simulink model "gm_parallel_min_cost_function_vopt_6phase"  (R2022a)
settings: Solver=FixedStepDiscrete  StartTime=0.0  StopTime=10.0  RelTol=1e-3
undefined symbols (not defined in the file or in its folder): f_c
libraries: hdlmdlgenlib x368
(part 3 of 3)

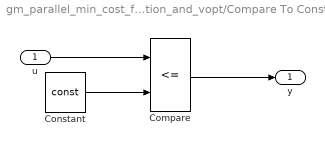
== system gm_parallel_min_cost_function_vopt_6phase/Min_cost_function_and_vopt/Compare To Constant ==
  u : Inport  OutDataTypeStr=int32  SampleTime=1e-08
  Compare : RelationalOperator  Operator=<=  OutDataTypeStr=boolean
  Constant : Constant  DisableCoverage=on  Value=const  OutDataTypeStr=Inherit: Inherit via back propagation  SampleTime=-1
  y : Outport  SampleTime=1e-08
  wires:
  u/1 -> Compare/1
  Compare/1 -> y/1
  Constant/1 -> Compare/2

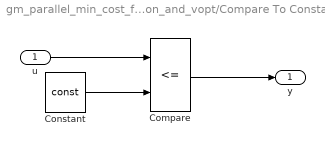
== system gm_parallel_min_cost_function_vopt_6phase/Min_cost_function_and_vopt/Compare To Constant1 ==
  u : Inport  OutDataTypeStr=fixdt(1, 33, 0)  SampleTime=1e-08
  Compare : RelationalOperator  Operator=<=  OutDataTypeStr=boolean
  Constant : Constant  DisableCoverage=on  Value=const  OutDataTypeStr=Inherit: Inherit via back propagation  SampleTime=-1
  y : Outport  SampleTime=1e-08
  wires:
  u/1 -> Compare/1
  Compare/1 -> y/1
  Constant/1 -> Compare/2

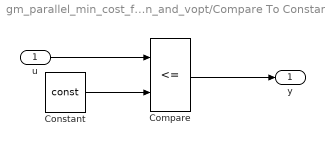
== system gm_parallel_min_cost_function_vopt_6phase/Min_cost_function_and_vopt/Compare To Constant10 ==
  u : Inport  OutDataTypeStr=fixdt(1, 33, 0)  SampleTime=1e-08
  Compare : RelationalOperator  Operator=<=  OutDataTypeStr=boolean
  Constant : Constant  DisableCoverage=on  Value=const  OutDataTypeStr=Inherit: Inherit via back propagation  SampleTime=-1
  y : Outport  SampleTime=1e-08
  wires:
  u/1 -> Compare/1
  Compare/1 -> y/1
  Constant/1 -> Compare/2

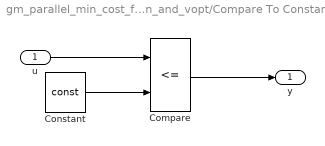
== system gm_parallel_min_cost_function_vopt_6phase/Min_cost_function_and_vopt/Compare To Constant11 ==
  u : Inport  OutDataTypeStr=fixdt(1, 33, 0)  SampleTime=1e-08
  Compare : RelationalOperator  Operator=<=  OutDataTypeStr=boolean
  Constant : Constant  DisableCoverage=on  Value=const  OutDataTypeStr=Inherit: Inherit via back propagation  SampleTime=-1
  y : Outport  SampleTime=1e-08
  wires:
  u/1 -> Compare/1
  Compare/1 -> y/1
  Constant/1 -> Compare/2

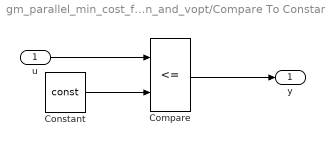
== system gm_parallel_min_cost_function_vopt_6phase/Min_cost_function_and_vopt/Compare To Constant12 ==
  u : Inport  OutDataTypeStr=fixdt(1, 33, 0)  SampleTime=1e-08
  Compare : RelationalOperator  Operator=<=  OutDataTypeStr=boolean
  Constant : Constant  DisableCoverage=on  Value=const  OutDataTypeStr=Inherit: Inherit via back propagation  SampleTime=-1
  y : Outport  SampleTime=1e-08
  wires:
  u/1 -> Compare/1
  Compare/1 -> y/1
  Constant/1 -> Compare/2

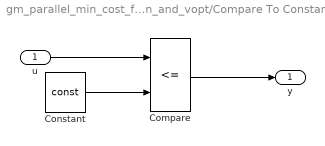
== system gm_parallel_min_cost_function_vopt_6phase/Min_cost_function_and_vopt/Compare To Constant13 ==
  u : Inport  OutDataTypeStr=fixdt(1, 33, 0)  SampleTime=1e-08
  Compare : RelationalOperator  Operator=<=  OutDataTypeStr=boolean
  Constant : Constant  DisableCoverage=on  Value=const  OutDataTypeStr=Inherit: Inherit via back propagation  SampleTime=-1
  y : Outport  SampleTime=1e-08
  wires:
  u/1 -> Compare/1
  Compare/1 -> y/1
  Constant/1 -> Compare/2

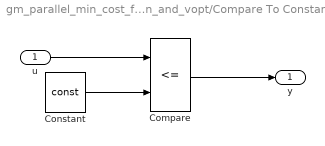
== system gm_parallel_min_cost_function_vopt_6phase/Min_cost_function_and_vopt/Compare To Constant14 ==
  u : Inport  OutDataTypeStr=fixdt(1, 33, 0)  SampleTime=1e-08
  Compare : RelationalOperator  Operator=<=  OutDataTypeStr=boolean
  Constant : Constant  DisableCoverage=on  Value=const  OutDataTypeStr=Inherit: Inherit via back propagation  SampleTime=-1
  y : Outport  SampleTime=1e-08
  wires:
  u/1 -> Compare/1
  Compare/1 -> y/1
  Constant/1 -> Compare/2

== system gm_parallel_min_cost_function_vopt_6phase/Min_cost_function_and_vopt/Compare To Constant15 ==
  u : Inport  OutDataTypeStr=fixdt(1, 33, 0)  SampleTime=1e-08
  Compare : RelationalOperator  Operator=<=  OutDataTypeStr=boolean
  Constant : Constant  DisableCoverage=on  Value=const  OutDataTypeStr=Inherit: Inherit via back propagation  SampleTime=-1
  y : Outport  SampleTime=1e-08
  wires:
  u/1 -> Compare/1
  Compare/1 -> y/1
  Constant/1 -> Compare/2

== system gm_parallel_min_cost_function_vopt_6phase/Min_cost_function_and_vopt/Compare To Constant2 ==
  u : Inport  OutDataTypeStr=fixdt(1, 33, 0)  SampleTime=1e-08
  Compare : RelationalOperator  Operator=<=  OutDataTypeStr=boolean
  Constant : Constant  DisableCoverage=on  Value=const  OutDataTypeStr=Inherit: Inherit via back propagation  SampleTime=-1
  y : Outport  SampleTime=1e-08
  wires:
  u/1 -> Compare/1
  Compare/1 -> y/1
  Constant/1 -> Compare/2

== system gm_parallel_min_cost_function_vopt_6phase/Min_cost_function_and_vopt/Compare To Constant3 ==
  u : Inport  OutDataTypeStr=fixdt(1, 33, 0)  SampleTime=1e-08
  Compare : RelationalOperator  Operator=<=  OutDataTypeStr=boolean
  Constant : Constant  DisableCoverage=on  Value=const  OutDataTypeStr=Inherit: Inherit via back propagation  SampleTime=-1
  y : Outport  SampleTime=1e-08
  wires:
  u/1 -> Compare/1
  Compare/1 -> y/1
  Constant/1 -> Compare/2

== system gm_parallel_min_cost_function_vopt_6phase/Min_cost_function_and_vopt/Compare To Constant4 ==
  u : Inport  OutDataTypeStr=fixdt(1, 33, 0)  SampleTime=1e-08
  Compare : RelationalOperator  Operator=<=  OutDataTypeStr=boolean
  Constant : Constant  DisableCoverage=on  Value=const  OutDataTypeStr=Inherit: Inherit via back propagation  SampleTime=-1
  y : Outport  SampleTime=1e-08
  wires:
  u/1 -> Compare/1
  Compare/1 -> y/1
  Constant/1 -> Compare/2

== system gm_parallel_min_cost_function_vopt_6phase/Min_cost_function_and_vopt/Compare To Constant5 ==
  u : Inport  OutDataTypeStr=fixdt(1, 33, 0)  SampleTime=1e-08
  Compare : RelationalOperator  Operator=<=  OutDataTypeStr=boolean
  Constant : Constant  DisableCoverage=on  Value=const  OutDataTypeStr=Inherit: Inherit via back propagation  SampleTime=-1
  y : Outport  SampleTime=1e-08
  wires:
  u/1 -> Compare/1
  Compare/1 -> y/1
  Constant/1 -> Compare/2

== system gm_parallel_min_cost_function_vopt_6phase/Min_cost_function_and_vopt/Compare To Constant6 ==
  u : Inport  OutDataTypeStr=fixdt(1, 33, 0)  SampleTime=1e-08
  Compare : RelationalOperator  Operator=<=  OutDataTypeStr=boolean
  Constant : Constant  DisableCoverage=on  Value=const  OutDataTypeStr=Inherit: Inherit via back propagation  SampleTime=-1
  y : Outport  SampleTime=1e-08
  wires:
  u/1 -> Compare/1
  Compare/1 -> y/1
  Constant/1 -> Compare/2

== system gm_parallel_min_cost_function_vopt_6phase/Min_cost_function_and_vopt/Compare To Constant7 ==
  u : Inport  OutDataTypeStr=fixdt(1, 33, 0)  SampleTime=1e-08
  Compare : RelationalOperator  Operator=<=  OutDataTypeStr=boolean
  Constant : Constant  DisableCoverage=on  Value=const  OutDataTypeStr=Inherit: Inherit via back propagation  SampleTime=-1
  y : Outport  SampleTime=1e-08
  wires:
  u/1 -> Compare/1
  Compare/1 -> y/1
  Constant/1 -> Compare/2

== system gm_parallel_min_cost_function_vopt_6phase/Min_cost_function_and_vopt/Compare To Constant8 ==
  u : Inport  OutDataTypeStr=fixdt(1, 33, 0)  SampleTime=1e-08
  Compare : RelationalOperator  Operator=<=  OutDataTypeStr=boolean
  Constant : Constant  DisableCoverage=on  Value=const  OutDataTypeStr=Inherit: Inherit via back propagation  SampleTime=-1
  y : Outport  SampleTime=1e-08
  wires:
  u/1 -> Compare/1
  Compare/1 -> y/1
  Constant/1 -> Compare/2

== system gm_parallel_min_cost_function_vopt_6phase/Min_cost_function_and_vopt/Compare To Constant9 ==
  u : Inport  OutDataTypeStr=fixdt(1, 33, 0)  SampleTime=1e-08
  Compare : RelationalOperator  Operator=<=  OutDataTypeStr=boolean
  Constant : Constant  DisableCoverage=on  Value=const  OutDataTypeStr=Inherit: Inherit via back propagation  SampleTime=-1
  y : Outport  SampleTime=1e-08
  wires:
  u/1 -> Compare/1
  Compare/1 -> y/1
  Constant/1 -> Compare/2

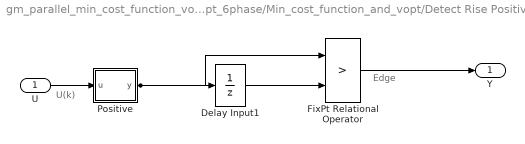
== system gm_parallel_min_cost_function_vopt_6phase/Min_cost_function_and_vopt/Detect Rise Positive ==
  note: Edge
  note: U(k)
  U : Inport  OutDataTypeStr=boolean  SampleTime=1e-08
  Delay Input1 : UnitDelay  Description=Store in Global RAM  DisableCoverage=on  InitialCondition=vinit  SampleTime=-1  HasFrameUpgradeWarning=on
  FixPt Relational Operator : RelationalOperator  Operator=>  OutDataTypeStr=boolean  ZeroCross=off  InputSameDT=off
  Positive : Subsystem  mask(Compare To Zero){relop=>, OutDataTypeStr=boolean, ZeroCross=off}
      mask prompts: relop "Simulink:masks:Operator_MP"; OutDataTypeStr "Simulink:masks:OutputDataType_MP"; ZeroCross "Simulink:masks:EnableZerocrossingDetection_MP"
      mask help: Simulink:masks:CompareToZero_MD
      mask init:
      | OutDataTypeStr = 'boolean';
      | ZeroCross = 'off';
      | blkName = 'parallel_min_cost_function_vopt_6phase/Min_cost_function_and_vopt/Detect Rise\nPositive/Positive';
      | relop = '>';
      | setValue = 'boolean';
      mask TypeOptions relop: == | ~= | < | <= | >= | >
      mask TypeOptions OutDataTypeStr: Simulink:masks:uint8 | Simulink:masks:boolean
      mask Callback ZeroCross: sl('zeroCrossEnable', gcbh);
      mask Display: disp([relop,' 0'])
  Y : Outport  SampleTime=1e-08
  wires:
  U/1 -> Positive/1(u)
  Delay Input1/1 -> FixPt Relational Operator/2
  FixPt Relational Operator/1 -> Y/1
  Positive/1(y) -> FixPt Relational Operator/1, Delay Input1/1

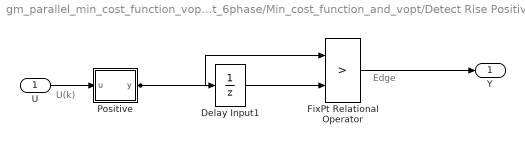
== system gm_parallel_min_cost_function_vopt_6phase/Min_cost_function_and_vopt/Detect Rise Positive1 ==
  note: Edge
  note: U(k)
  U : Inport  OutDataTypeStr=boolean  SampleTime=1e-08
  Delay Input1 : UnitDelay  Description=Store in Global RAM  DisableCoverage=on  InitialCondition=vinit  SampleTime=-1  HasFrameUpgradeWarning=on
  FixPt Relational Operator : RelationalOperator  Operator=>  OutDataTypeStr=boolean  ZeroCross=off  InputSameDT=off
  Positive : Subsystem  mask(Compare To Zero){relop=>, OutDataTypeStr=boolean, ZeroCross=off}
      mask prompts: relop "Simulink:masks:Operator_MP"; OutDataTypeStr "Simulink:masks:OutputDataType_MP"; ZeroCross "Simulink:masks:EnableZerocrossingDetection_MP"
      mask help: Simulink:masks:CompareToZero_MD
      mask init:
      | OutDataTypeStr = 'boolean';
      | ZeroCross = 'off';
      | blkName = 'parallel_min_cost_function_vopt_6phase/Min_cost_function_and_vopt/Detect Rise\nPositive1/Positive';
      | relop = '>';
      | setValue = 'boolean';
      mask TypeOptions relop: == | ~= | < | <= | >= | >
      mask TypeOptions OutDataTypeStr: Simulink:masks:uint8 | Simulink:masks:boolean
      mask Callback ZeroCross: sl('zeroCrossEnable', gcbh);
      mask Display: disp([relop,' 0'])
  Y : Outport  SampleTime=1e-08
  wires:
  U/1 -> Positive/1(u)
  Delay Input1/1 -> FixPt Relational Operator/2
  FixPt Relational Operator/1 -> Y/1
  Positive/1(y) -> FixPt Relational Operator/1, Delay Input1/1

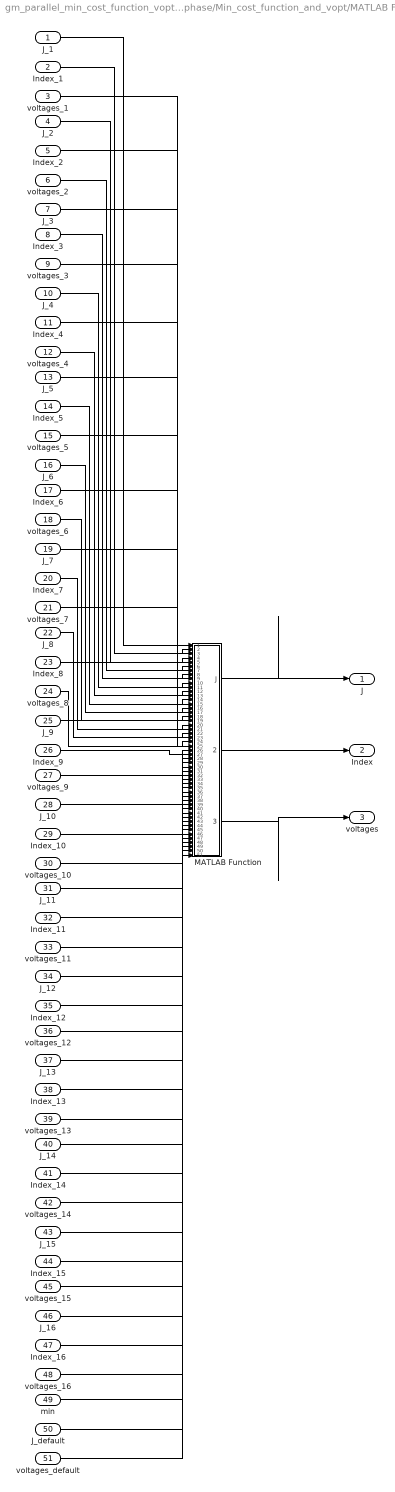
== system gm_parallel_min_cost_function_vopt_6phase/Min_cost_function_and_vopt/MATLAB Function ==
  J_1 : Inport  OutDataTypeStr=fixdt(1, 20, 11)  PortDimensions=1  SampleTime=1e-08
  Index_1 : Inport  Port=2  OutDataTypeStr=int32  PortDimensions=1  SampleTime=1e-08
  voltages_1 : Inport  Port=3  OutDataTypeStr=fixdt(1, 24, 11)  PortDimensions=[4]  SampleTime=1e-08
  J_2 : Inport  Port=4  OutDataTypeStr=fixdt(1, 20, 11)  PortDimensions=1  SampleTime=1e-08
  Index_2 : Inport  Port=5  OutDataTypeStr=int32  PortDimensions=1  SampleTime=1e-08
  voltages_2 : Inport  Port=6  OutDataTypeStr=fixdt(1, 24, 11)  PortDimensions=[4]  SampleTime=1e-08
  J_3 : Inport  Port=7  OutDataTypeStr=fixdt(1, 20, 11)  PortDimensions=1  SampleTime=1e-08
  Index_3 : Inport  Port=8  OutDataTypeStr=int32  PortDimensions=1  SampleTime=1e-08
  voltages_3 : Inport  Port=9  OutDataTypeStr=fixdt(1, 24, 11)  PortDimensions=[4]  SampleTime=1e-08
  J_4 : Inport  Port=10  OutDataTypeStr=fixdt(1, 20, 11)  PortDimensions=1  SampleTime=1e-08
  Index_4 : Inport  Port=11  OutDataTypeStr=int32  PortDimensions=1  SampleTime=1e-08
  voltages_4 : Inport  Port=12  OutDataTypeStr=fixdt(1, 24, 11)  PortDimensions=[4]  SampleTime=1e-08
  J_5 : Inport  Port=13  OutDataTypeStr=fixdt(1, 20, 11)  PortDimensions=1  SampleTime=1e-08
  Index_5 : Inport  Port=14  OutDataTypeStr=int32  PortDimensions=1  SampleTime=1e-08
  voltages_5 : Inport  Port=15  OutDataTypeStr=fixdt(1, 24, 11)  PortDimensions=[4]  SampleTime=1e-08
  J_6 : Inport  Port=16  OutDataTypeStr=fixdt(1, 20, 11)  PortDimensions=1  SampleTime=1e-08
  Index_6 : Inport  Port=17  OutDataTypeStr=int32  PortDimensions=1  SampleTime=1e-08
  voltages_6 : Inport  Port=18  OutDataTypeStr=fixdt(1, 24, 11)  PortDimensions=[4]  SampleTime=1e-08
  J_7 : Inport  Port=19  OutDataTypeStr=fixdt(1, 20, 11)  PortDimensions=1  SampleTime=1e-08
  Index_7 : Inport  Port=20  OutDataTypeStr=int32  PortDimensions=1  SampleTime=1e-08
  voltages_7 : Inport  Port=21  OutDataTypeStr=fixdt(1, 24, 11)  PortDimensions=[4]  SampleTime=1e-08
  J_8 : Inport  Port=22  OutDataTypeStr=fixdt(1, 20, 11)  PortDimensions=1  SampleTime=1e-08
  Index_8 : Inport  Port=23  OutDataTypeStr=int32  PortDimensions=1  SampleTime=1e-08
  voltages_8 : Inport  Port=24  OutDataTypeStr=fixdt(1, 24, 11)  PortDimensions=[4]  SampleTime=1e-08
  J_9 : Inport  Port=25  OutDataTypeStr=fixdt(1, 20, 11)  PortDimensions=1  SampleTime=1e-08
  Index_9 : Inport  Port=26  OutDataTypeStr=int32  PortDimensions=1  SampleTime=1e-08
  voltages_9 : Inport  Port=27  OutDataTypeStr=fixdt(1, 24, 11)  PortDimensions=[4]  SampleTime=1e-08
  J_10 : Inport  Port=28  OutDataTypeStr=fixdt(1, 20, 11)  PortDimensions=1  SampleTime=1e-08
  Index_10 : Inport  Port=29  OutDataTypeStr=int32  PortDimensions=1  SampleTime=1e-08
  voltages_10 : Inport  Port=30  OutDataTypeStr=fixdt(1, 24, 11)  PortDimensions=[4]  SampleTime=1e-08
  J_11 : Inport  Port=31  OutDataTypeStr=fixdt(1, 20, 11)  PortDimensions=1  SampleTime=1e-08
  Index_11 : Inport  Port=32  OutDataTypeStr=int32  PortDimensions=1  SampleTime=1e-08
  voltages_11 : Inport  Port=33  OutDataTypeStr=fixdt(1, 24, 11)  PortDimensions=[4]  SampleTime=1e-08
  J_12 : Inport  Port=34  OutDataTypeStr=fixdt(1, 20, 11)  PortDimensions=1  SampleTime=1e-08
  Index_12 : Inport  Port=35  OutDataTypeStr=int32  PortDimensions=1  SampleTime=1e-08
  voltages_12 : Inport  Port=36  OutDataTypeStr=fixdt(1, 24, 11)  PortDimensions=[4]  SampleTime=1e-08
  J_13 : Inport  Port=37  OutDataTypeStr=fixdt(1, 20, 11)  PortDimensions=1  SampleTime=1e-08
  Index_13 : Inport  Port=38  OutDataTypeStr=int32  PortDimensions=1  SampleTime=1e-08
  voltages_13 : Inport  Port=39  OutDataTypeStr=fixdt(1, 24, 11)  PortDimensions=[4]  SampleTime=1e-08
  J_14 : Inport  Port=40  OutDataTypeStr=fixdt(1, 20, 11)  PortDimensions=1  SampleTime=1e-08
  Index_14 : Inport  Port=41  OutDataTypeStr=int32  PortDimensions=1  SampleTime=1e-08
  voltages_14 : Inport  Port=42  OutDataTypeStr=fixdt(1, 24, 11)  PortDimensions=[4]  SampleTime=1e-08
  J_15 : Inport  Port=43  OutDataTypeStr=fixdt(1, 20, 11)  PortDimensions=1  SampleTime=1e-08
  Index_15 : Inport  Port=44  OutDataTypeStr=int32  PortDimensions=1  SampleTime=1e-08
  voltages_15 : Inport  Port=45  OutDataTypeStr=fixdt(1, 24, 11)  PortDimensions=[4]  SampleTime=1e-08
  J_16 : Inport  Port=46  OutDataTypeStr=fixdt(1, 20, 11)  PortDimensions=1  SampleTime=1e-08
  Index_16 : Inport  Port=47  OutDataTypeStr=int32  PortDimensions=1  SampleTime=1e-08
  voltages_16 : Inport  Port=48  OutDataTypeStr=fixdt(1, 24, 11)  PortDimensions=[4]  SampleTime=1e-08
  min : Inport  Port=49  OutDataTypeStr=fixdt(1, 20, 11)  PortDimensions=1  SampleTime=1e-08
  J_default : Inport  Port=50  OutDataTypeStr=fixdt(1, 20, 11)  PortDimensions=1  SampleTime=1e-08
  voltages_default : Inport  Port=51  OutDataTypeStr=fixdt(1, 24, 11)  PortDimensions=[4]  SampleTime=1e-08
  MATLAB Function : MATLAB Function  TreatAsAtomicUnit=on
  J : Outport  SampleTime=1e-08  VectorParamsAs1DForOutWhenUnconnected=off
  Index : Outport  Port=2  SampleTime=1e-08
  voltages : Outport  Port=3  SampleTime=1e-08
  wires:
  J_1/1 -> MATLAB Function/1(J_1)
  Index_1/1 -> MATLAB Function/2(Index_1)
  voltages_1/1 -> MATLAB Function/3(voltages_1)
  J_2/1 -> MATLAB Function/4(J_2)
  Index_2/1 -> MATLAB Function/5(Index_2)
  voltages_2/1 -> MATLAB Function/6(voltages_2)
  J_3/1 -> MATLAB Function/7(J_3)
  Index_3/1 -> MATLAB Function/8(Index_3)
  voltages_3/1 -> MATLAB Function/9(voltages_3)
  J_4/1 -> MATLAB Function/10(J_4)
  Index_4/1 -> MATLAB Function/11(Index_4)
  voltages_4/1 -> MATLAB Function/12(voltages_4)
  J_5/1 -> MATLAB Function/13(J_5)
  Index_5/1 -> MATLAB Function/14(Index_5)
  voltages_5/1 -> MATLAB Function/15(voltages_5)
  J_6/1 -> MATLAB Function/16(J_6)
  Index_6/1 -> MATLAB Function/17(Index_6)
  voltages_6/1 -> MATLAB Function/18(voltages_6)
  J_7/1 -> MATLAB Function/19(J_7)
  Index_7/1 -> MATLAB Function/20(Index_7)
  voltages_7/1 -> MATLAB Function/21(voltages_7)
  J_8/1 -> MATLAB Function/22(J_8)
  Index_8/1 -> MATLAB Function/23(Index_8)
  voltages_8/1 -> MATLAB Function/24(voltages_8)
  J_9/1 -> MATLAB Function/25(J_9)
  Index_9/1 -> MATLAB Function/26(Index_9)
  voltages_9/1 -> MATLAB Function/27(voltages_9)
  J_10/1 -> MATLAB Function/28(J_10)
  Index_10/1 -> MATLAB Function/29(Index_10)
  voltages_10/1 -> MATLAB Function/30(voltages_10)
  J_11/1 -> MATLAB Function/31(J_11)
  Index_11/1 -> MATLAB Function/32(Index_11)
  voltages_11/1 -> MATLAB Function/33(voltages_11)
  J_12/1 -> MATLAB Function/34(J_12)
  Index_12/1 -> MATLAB Function/35(Index_12)
  voltages_12/1 -> MATLAB Function/36(voltages_12)
  J_13/1 -> MATLAB Function/37(J_13)
  Index_13/1 -> MATLAB Function/38(Index_13)
  voltages_13/1 -> MATLAB Function/39(voltages_13)
  J_14/1 -> MATLAB Function/40(J_14)
  Index_14/1 -> MATLAB Function/41(Index_14)
  voltages_14/1 -> MATLAB Function/42(voltages_14)
  J_15/1 -> MATLAB Function/43(J_15)
  Index_15/1 -> MATLAB Function/44(Index_15)
  voltages_15/1 -> MATLAB Function/45(voltages_15)
  J_16/1 -> MATLAB Function/46(J_16)
  Index_16/1 -> MATLAB Function/47(Index_16)
  voltages_16/1 -> MATLAB Function/48(voltages_16)
  min/1 -> MATLAB Function/49(min)
  J_default/1 -> MATLAB Function/50(J_default)
  voltages_default/1 -> MATLAB Function/51(voltages_default)
  MATLAB Function/1(J) -> J/1
  MATLAB Function/2(Index) -> Index/1
  MATLAB Function/3(voltages) -> voltages/1

== system gm_parallel_min_cost_function_vopt_6phase/Min_cost_function_and_vopt/Detect Rise Positive/Positive ==
  u : Inport  OutDataTypeStr=boolean  SampleTime=1e-08
  Compare : RelationalOperator  Operator=>  OutDataTypeStr=boolean  ZeroCross=off
  Constant : Constant  DisableCoverage=on  Value=0  OutDataTypeStr=Inherit: Inherit via back propagation  SampleTime=-1  PreserveConstantTs=on
  y : Outport  SampleTime=1e-08
  wires:
  u/1 -> Compare/1
  Compare/1 -> y/1
  Constant/1 -> Compare/2

== system gm_parallel_min_cost_function_vopt_6phase/Min_cost_function_and_vopt/Detect Rise Positive1/Positive ==
  u : Inport  OutDataTypeStr=boolean  SampleTime=1e-08
  Compare : RelationalOperator  Operator=>  OutDataTypeStr=boolean  ZeroCross=off
  Constant : Constant  DisableCoverage=on  Value=0  OutDataTypeStr=Inherit: Inherit via back propagation  SampleTime=-1  PreserveConstantTs=on
  y : Outport  SampleTime=1e-08
  wires:
  u/1 -> Compare/1
  Compare/1 -> y/1
  Constant/1 -> Compare/2

== matlab function gm_parallel_min_cost_function_vopt_6phase/Min_cost_function_and_vopt/MATLAB Function/MATLAB Function ==
  data: J_1 input; Index_1 input; J output fixdt(1,20,11); voltages_1 input; J_2 input; Index_2 input; voltages_2 input; J_3 input; Index_3 input; voltages_3 input; J_4 input; Index_4 input; voltages_4 input; J_5 input; Index_5 input; voltages_5 input; J_6 input; Index_6 input; voltages_6 input; J_7 input; Index_7 input; voltages_7 input; J_8 input; Index_8 input; voltages_8 input; J_9 input; Index_9 input; voltages_9 input; J_10 input; Index_10 input; voltages_10 input; J_11 input; Index_11 input; voltages_11 input; J_12 input; Index_12 input; voltages_12 input; J_13 input; Index_13 input; voltages_13 input; J_14 input; Index_14 input; voltages_14 input; J_15 input; Index_15 input; voltages_15 input; J_16 input; Index_16 input; voltages_16 input; Index output int32; min input fixdt(1,20,11); J_default input; voltages output; voltages_default input
function [J, Index, voltages] = fcn(J_1, Index_1, voltages_1, J_2, Index_2, voltages_2, J_3, Index_3, voltages_3, J_4, Index_4, voltages_4, J_5, Index_5, voltages_5, J_6, Index_6, voltages_6, ...
                                    J_7, Index_7, voltages_7, J_8, Index_8, voltages_8, J_9, Index_9, voltages_9, J_10, Index_10, voltages_10, J_11, Index_11, voltages_11, J_12, Index_12, voltages_12, ...
                                    J_13, Index_13, voltages_13, J_14, Index_14, voltages_14, J_15, Index_15, voltages_15, J_16, Index_16, voltages_16, min, J_default,voltages_default)



if J_1 == min
    Index = Index_1;
    voltages = voltages_1;
    J = J_1;
elseif J_2 == min
    Index = Index_2;
    voltages = voltages_2;
    J = J_2;
elseif J_3 == min
    Index = Index_3;
    voltages = voltages_3;
    J = J_3;
elseif J_4 == min
    Index = Index_4;
    voltages = voltages_4;
    J = J_4;
elseif J_5 == min
    Index = Index_5;
    voltages = voltages_5;
    J = J_5;
elseif J_6 == min
    Index = Index_6;
    voltages = voltages_6;
    J = J_6;
elseif J_7 == min
    Index = Index_7;
    voltages = voltages_7;
    J = J_7;
elseif J_8 == min
    Index = Index_8;
    voltages = voltages_8;
    J = J_8;
elseif J_9 == min
    Index = Index_9;
    voltages = voltages_9;
    J = J_9;
elseif J_10 == min
    Index = Index_10;
    voltages = voltages_10;
    J = J_10;
elseif J_11 == min
    Index = Index_11;
    voltages = voltages_11;
    J = J_11;
elseif J_12 == min
    Index = Index_12;
    voltages = voltages_12;
    J = J_12;
elseif J_13 == min
    Index = Index_13;
    voltages = voltages_13;
    J = J_13;
elseif J_14 == min
    Index = Index_14;
    voltages = voltages_14;
    J = J_14;
elseif J_15 == min
    Index = Index_15;
    voltages = voltages_15;
    J = J_15;
elseif J_16 == min
    Index = Index_16;
    voltages = voltages_16;
    J = J_16;
else 
    Index = int32(0);
    J = J_default;
    voltages = voltages_default;
end
